simulink model "start_training"  (R2023b)
settings: Solver=FixedStepAuto  StartTime=0.0  StopTime=10  RelTol=1e-3
libraries: instrumentlib x2
settings Model: PacingRate=0.089000  Creator=pc  LastModifiedBy=pc

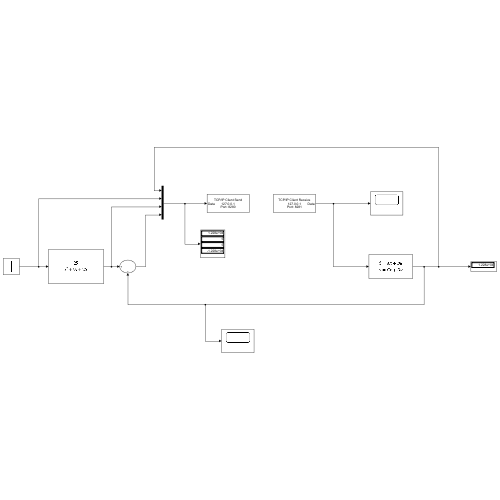
[thumbnail: Simulink's stored preview of the top-level diagram]
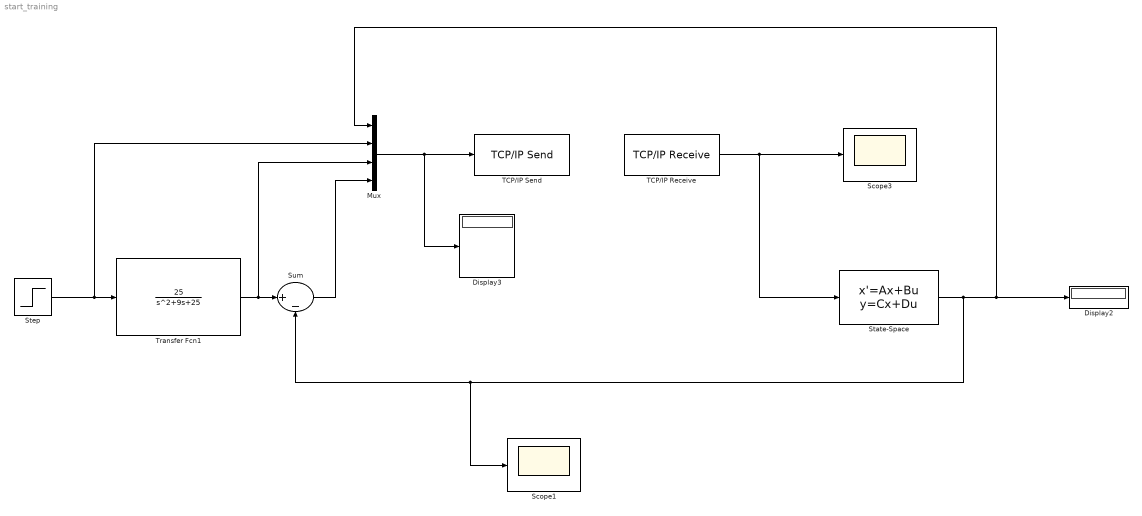
== system start_training ==
  Display2 : Display
  Display3 : Display
  Mux : Mux
  Scope1 : Scope
  Scope3 : Scope
  State-Space : StateSpace  D=0  InitialCondition=0  ContinuousStateAttributes='Controlled_Object'
  Step : Step  Before=5  After=5  SampleTime=0
  Sum : Sum  Inputs=|+-
  TCP/IP Receive : instrumentlib/TCP//IP Receive  Host=127.0.0.1  Port=8281  DataSize=[1]  DataType=double  ASCIIFormatting=%f  Terminator=LF  CustomTerminator=10  ByteOrder=big-endian  EnableBlockingMode=on  Timeout=10  SampleTime=0.01  SimulateUsing=Interpreted execution
  TCP/IP Send : instrumentlib/TCP//IP Send  Host=127.0.0.1  Port=8280  ByteOrder=big-endian  EnableBlockingMode=on  Timeout=10  TransferDelay=on  SimulateUsing=Interpreted execution
  Transfer Fcn1 : TransferFcn  Numerator=[25]  Denominator=[1 9 25]  ContinuousStateAttributes='Reference_Model'
  wires:
  Sum/1 -> Mux/4
  Transfer Fcn1/1 -> Mux/3, Sum/1
  Step/1 -> Mux/2, Transfer Fcn1/1
  TCP/IP Receive/1 -> State-Space/1, Scope3/1
  Mux/1 -> Display3/1, TCP/IP Send/1
  State-Space/1 -> Scope1/1, Sum/2, Mux/1, Display2/1
